simulink model "Tricopter_Controlled_development"  (R2015a)
settings: Solver=ode2  SolverMode=SingleTasking  StartTime=0.0  StopTime=inf  FixedStep=T_sim  RelTol=1e-3
values from neighbouring files (symbols this model uses):
  A_l_max_x = sqrt( (A_z_max)^2  -  g^2  )    [Run3Copter.m]
  A_l_max_y = g*tand(15)    [Run3Copter.m]
  A_x = 0.015    [SetupComplete.m]
  A_y = A_x    (= 0.015)    [SetupComplete.m]
  A_z = 0.16    [SetupComplete.m]
  A_z_max = Max_Thrust*3/m    [Run3Copter.m]
  Alt_0 = input(' Give the initial altitude (m): ')    [Run3Copter.m]
  C_x = 1.2    [SetupComplete.m]
  C_y = C_x    (= 1.2)    [SetupComplete.m]
  C_z = 2.2    [SetupComplete.m]
  CG_0 = [0,0,0.02]'    [SetupComplete.m]
  epsilon = 0.01    [Run3Copter.m]
  eta_23 = deg2rad(-1.3)    [Run3Copter.m]
  g = 9.81    [SetupComplete.m]
  h = 0.08    [SetupComplete.m]
  h_M = 0.064    [SetupComplete.m]
  I_BAC_0 = [ Ix,0,Ixz;0,Iy,0;Ixz,0,Iz]    [SetupComplete.m]
  Initial_Omegas = Omega_hover    [Run3Copter.m]
  Initial_Torques = Torque_hover    [Run3Copter.m]
  Ix = 0.103    [SetupComplete.m]
  Iy = 0.147    [SetupComplete.m]
  Iz = 0.237    [SetupComplete.m]
  l = 0.345    [SetupComplete.m]
  l_arm = 0.264    [SetupComplete.m]
  latitude = 52.071118    [Run3Copter.m]
  longitude = -0.627404    [Run3Copter.m]
  m = 3.51    [SetupComplete.m]
  m_0 = 2.61    [SetupComplete.m]
  m_M = 0.300    (= 0.3)    [SetupComplete.m]
  rho = 1.15    [SetupComplete.m]
  Rotation_sign = [ 1,-1,-1]    [SetupComplete.m]
  T_ctrl = 0.02    [Run3Copter.m]
  T_sim = 0.01    [Run3Copter.m]
  throtle_1 = 0*0.745    (= 0)    [Run3Copter.m]
  throtle_23 = throtle_1/cos(eta_23)    [Run3Copter.m]
  v_i0 = sqrt( 1/3*m*g/(2*rho*pi*R^2)  )    [SetupComplete.m]
undefined symbols (not defined in the file or in its folder): DOWN_0, EAST_0, Newton, NORTH_0, P_0, Q_0, R_0, Raphson, U_0, V_0, W_0
libraries: Adaptive_FaultTolerantControl x30, XXCopter_Control x23, simulink_extras x17, XXCopter x5, simulink x2, qcatlib x1, XXCopter_C x1
(part 3 of 4)

== system Tricopter_Controlled_development/TriCopter FCS development/Inner Controller/PI Controller/keep -pi//pi2 ==
  in (rad) : Inport
  Constant : Constant  Value=180
  Constant2 : Constant  Value=360
  Gain : Gain  Gain=360
  Math Function2 : Math  Operator=rem  SaturateOnIntegerOverflow=on
  Product : Product  Inputs=*/  RndMeth=Zero
  Rounding Function : Rounding  Operator=fix
  Sum2 : Sum  Inputs=|-+
  deg2rad1 : Gain  Gain=pi/180  SaturateOnIntegerOverflow=on  OutDataTypeStr=Inherit: Same as input  ParamDataTypeStr=Inherit: Same as input
  rad2deg : Gain  Gain=180/pi  SaturateOnIntegerOverflow=on  OutDataTypeStr=Inherit: Same as input  ParamDataTypeStr=Inherit: Same as input
  out (rad) : Outport
  wires:
  deg2rad1/1 -> out (rad)/1
  Sum2/1 -> deg2rad1/1
  Math Function2/1 -> Sum2/2, Product/1
  Constant2/1 -> Math Function2/2
  rad2deg/1 -> Math Function2/1
  Gain/1 -> Sum2/1
  Rounding Function/1 -> Gain/1
  Product/1 -> Rounding Function/1
  Constant/1 -> Product/2
  in (rad)/1 -> rad2deg/1

== system Tricopter_Controlled_development/TriCopter FCS development/Inner Controller/PI Controller/keep -pi//pi3 ==
  in (rad) : Inport
  Constant : Constant  Value=180
  Constant2 : Constant  Value=360
  Gain : Gain  Gain=360
  Math Function2 : Math  Operator=rem  SaturateOnIntegerOverflow=on
  Product : Product  Inputs=*/  RndMeth=Zero
  Rounding Function : Rounding  Operator=fix
  Sum2 : Sum  Inputs=|-+
  deg2rad1 : Gain  Gain=pi/180  SaturateOnIntegerOverflow=on  OutDataTypeStr=Inherit: Same as input  ParamDataTypeStr=Inherit: Same as input
  rad2deg : Gain  Gain=180/pi  SaturateOnIntegerOverflow=on  OutDataTypeStr=Inherit: Same as input  ParamDataTypeStr=Inherit: Same as input
  out (rad) : Outport
  wires:
  in (rad)/1 -> rad2deg/1
  Constant/1 -> Product/2
  Product/1 -> Rounding Function/1
  Rounding Function/1 -> Gain/1
  Gain/1 -> Sum2/1
  rad2deg/1 -> Math Function2/1
  Constant2/1 -> Math Function2/2
  Math Function2/1 -> Product/1, Sum2/2
  Sum2/1 -> deg2rad1/1
  deg2rad1/1 -> out (rad)/1

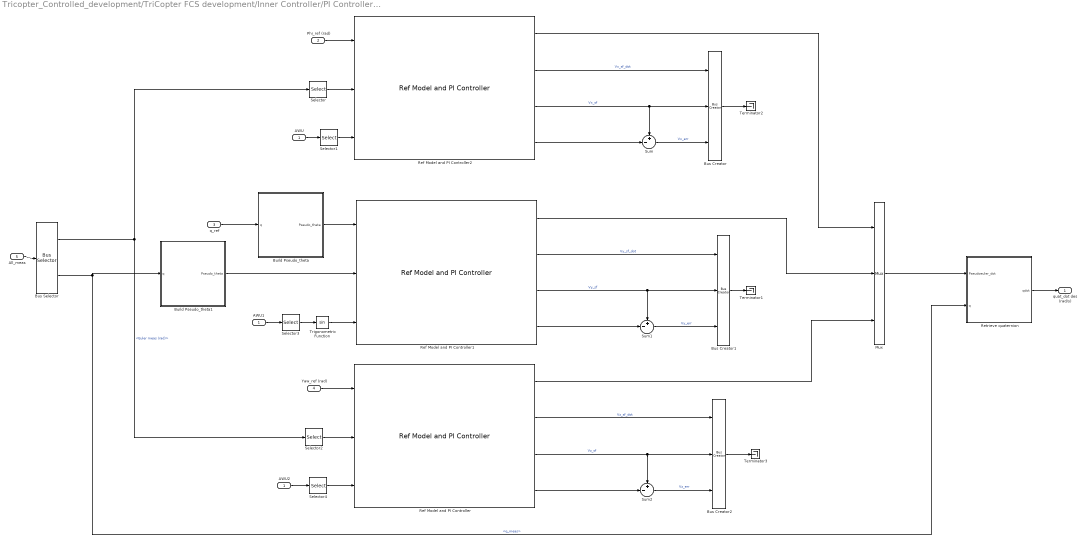
== system Tricopter_Controlled_development/TriCopter FCS development/Inner Controller/PI Controller Quaternions/Attitude Controller ==
  AWU : Inport
  Phi_ref (rad) : Inport  Port=2
  q_ref : Inport  Port=3
  Yaw_ref (rad) : Inport  Port=4
  All_meas : Inport  Port=5
  AWU1 : InportShadow
  AWU2 : InportShadow
  Build Pseudo_theta : MATLAB Function  TreatAsAtomicUnit=on
  Build Pseudo_theta1 : MATLAB Function  TreatAsAtomicUnit=on
  Bus Creator : BusCreator  Inputs=3
  Bus Creator1 : BusCreator  Inputs=3
  Bus Creator2 : BusCreator  Inputs=3
  Bus Selector : BusSelector  OutputSignals=Meas.Euler meas (rad),Meas.q_meas
  Mux : Mux  Inputs=3
  Ref Model and PI Controller : Adaptive_FaultTolerantControl/Ref Model and PI Controller  delta=0  tau=2  y_i=0  K_f=0  K_a=1  Con_way=pro  omega_n=4  xi=0.5  Z1=-30  K_b=2  f_i=0.15  f_c=1
  Ref Model and PI Controller1 : Adaptive_FaultTolerantControl/Ref Model and PI Controller  delta=0  tau=1.5  y_i=0  K_f=0  K_a=1  Con_way=pro  omega_n=4  xi=0.5  Z1=-30  K_b=1.2  f_i=0.1  f_c=1
  Ref Model and PI Controller2 : Adaptive_FaultTolerantControl/Ref Model and PI Controller  delta=0  tau=1.5  y_i=0  K_f=0  K_a=1  Con_way=pro  omega_n=4  xi=0.5  Z1=-30  K_b=1.5  f_i=0.1  f_c=1
  Retrieve quaternion : MATLAB Function  TreatAsAtomicUnit=on
  Selector : Selector  InputPortWidth=3
  Selector1 : Selector  InputPortWidth=3
  Selector2 : Selector  InputPortWidth=3  Indices=3
  Selector3 : Selector  InputPortWidth=3  Indices=2
  Selector4 : Selector  InputPortWidth=3  Indices=3
  Sum : Sum  Inputs=+-|
  Sum1 : Sum  Inputs=+-|
  Sum2 : Sum  Inputs=+-|
  Terminator1 : Terminator
  Terminator2 : Terminator
  Terminator3 : Terminator
  Trigonometric Function : Trigonometry
  quat_dot des (rad/s) : Outport
  wires:
  Ref Model and PI Controller/4 -> Sum2/2
  Sum2/1 -> Bus Creator2/3  "Vz_err"
  Ref Model and PI Controller/3 -> Bus Creator2/2, Sum2/1  "Vz_sf"
  Ref Model and PI Controller/2 -> Bus Creator2/1  "Vz_sf_dot"
  Ref Model and PI Controller1/4 -> Sum1/2
  Sum1/1 -> Bus Creator1/3  "Vy_err"
  Ref Model and PI Controller1/3 -> Bus Creator1/2, Sum1/1  "Vy_sf"
  Ref Model and PI Controller1/2 -> Bus Creator1/1  "Vy_sf_dot"
  Ref Model and PI Controller2/4 -> Sum/2
  Bus Creator2/1 -> Terminator3/1
  Bus Creator1/1 -> Terminator1/1
  Bus Creator/1 -> Terminator2/1
  Sum/1 -> Bus Creator/3  "Vx_err"
  Ref Model and PI Controller2/3 -> Bus Creator/2, Sum/1  "Vx_sf"
  Ref Model and PI Controller2/2 -> Bus Creator/1  "Vx_sf_dot"
  Yaw_ref (rad)/1 -> Ref Model and PI Controller/1
  Selector/1 -> Ref Model and PI Controller2/2
  Bus Selector/2 -> Retrieve quaternion/2(q), Build Pseudo_theta1/1(q)  "<q_meas>"
  All_meas/1 -> Bus Selector/1
  q_ref/1 -> Build Pseudo_theta/1(q)
  Phi_ref (rad)/1 -> Ref Model and PI Controller2/1
  Retrieve quaternion/1(qdot) -> quat_dot des (rad/s)/1
  Ref Model and PI Controller2/1 -> Mux/1
  Ref Model and PI Controller/1 -> Mux/3
  Ref Model and PI Controller1/1 -> Mux/2
  Mux/1 -> Retrieve quaternion/1(Pseudoeuler_dot)
  Selector2/1 -> Ref Model and PI Controller/2
  Bus Selector/1 -> Selector2/1, Selector/1  "<Euler meas (rad)>"
  Build Pseudo_theta1/1(Pseudo_theta) -> Ref Model and PI Controller1/2
  Build Pseudo_theta/1(Pseudo_theta) -> Ref Model and PI Controller1/1
  Selector1/1 -> Ref Model and PI Controller2/3
  AWU/1 -> Selector1/1
  AWU1/1 -> Selector3/1
  AWU2/1 -> Selector4/1
  Selector4/1 -> Ref Model and PI Controller/3
  Selector3/1 -> Trigonometric Function/1
  Trigonometric Function/1 -> Ref Model and PI Controller1/3

== system Tricopter_Controlled_development/TriCopter FCS development/Inner Controller/PI Controller Quaternions/Body Rates Controller ==
  p_ref : Inport
  q_ref : Inport  Port=2
  r_ref : Inport  Port=3
  All_meas : Inport  Port=4
  Bus Creator : BusCreator
  Bus Creator1 : BusCreator
  Bus Creator2 : BusCreator
  Bus Selector : BusSelector  OutputSignals=Meas.omega_b meas (rad/s)
  Mux : Mux  Inputs=3
  Ref Model and P Controller p : Adaptive_FaultTolerantControl/Ref Model and P Controller  tau=0.7  y_i=0  K_f=0.7  K_b=6
  Ref Model and P Controller q : Adaptive_FaultTolerantControl/Ref Model and P Controller  tau=0.7  y_i=0  K_f=0.7  K_b=6
  Ref Model and P Controller r : Adaptive_FaultTolerantControl/Ref Model and P Controller  tau=1.5  y_i=0  K_f=0.7  K_b=1.5
  Selector : Selector  InputPortWidth=3
  Selector1 : Selector  InputPortWidth=3  Indices=2
  Selector2 : Selector  InputPortWidth=3  Indices=3
  Sum : Sum  Inputs=+-|
  Sum1 : Sum  Inputs=+-|
  Sum2 : Sum  Inputs=+-|
  Terminator1 : Terminator
  Terminator2 : Terminator
  Terminator3 : Terminator
  Angular acc des (rad/s^2) : Outport
  wires:
  Ref Model and P Controller r/5 -> Bus Creator2/4  "K_b_r"
  Ref Model and P Controller r/4 -> Sum2/2
  Sum2/1 -> Bus Creator2/3  "r_err"
  Ref Model and P Controller r/3 -> Bus Creator2/2, Sum2/1  "r_sf"
  Ref Model and P Controller r/2 -> Bus Creator2/1  "r_sf_dot"
  Ref Model and P Controller q/5 -> Bus Creator1/4  "K_b_q"
  Ref Model and P Controller q/4 -> Sum1/2
  Sum1/1 -> Bus Creator1/3  "q_err"
  Ref Model and P Controller q/3 -> Bus Creator1/2, Sum1/1  "q_sf"
  Ref Model and P Controller q/2 -> Bus Creator1/1  "q_sf_dot"
  Ref Model and P Controller p/5 -> Bus Creator/4  "K_b_p"
  Ref Model and P Controller p/4 -> Sum/2
  Selector2/1 -> Ref Model and P Controller r/2
  Bus Creator2/1 -> Terminator3/1
  Bus Creator1/1 -> Terminator1/1
  Bus Creator/1 -> Terminator2/1
  Sum/1 -> Bus Creator/3  "p_err"
  Ref Model and P Controller p/3 -> Bus Creator/2, Sum/1  "p_sf"
  Ref Model and P Controller p/2 -> Bus Creator/1  "p_sf_dot"
  r_ref/1 -> Ref Model and P Controller r/1
  Selector1/1 -> Ref Model and P Controller q/2
  q_ref/1 -> Ref Model and P Controller q/1
  Mux/1 -> Angular acc des (rad/s^2)/1
  Selector/1 -> Ref Model and P Controller p/2
  p_ref/1 -> Ref Model and P Controller p/1
  Bus Selector/1 -> Selector2/1, Selector1/1, Selector/1  "<omega_b meas (rad/s)>"
  All_meas/1 -> Bus Selector/1
  Ref Model and P Controller r/1 -> Mux/3
  Ref Model and P Controller q/1 -> Mux/2
  Ref Model and P Controller p/1 -> Mux/1

== system Tricopter_Controlled_development/TriCopter FCS development/Inner Controller/PI Controller Quaternions/Limits in Ang accel ==
  note: Here it is assumed that at all time every prop is generating m*g/3 newtons of force . It is conservative?
  Ang Ace des : Inport
  Euler meas : Inport  Port=2
  Limis eval : MATLAB Function  TreatAsAtomicUnit=on
  Saturation Dynamic : simulink/Discontinuities/Saturation Dynamic  OutMin=[]  OutMax=[]  OutDataTypeStr=Inherit: Same as second input  OutDataType=fixdt(1, 16)  OutScaling=2^-10  DoSatur=off
  ang Ace des : Outport
  wires:
  Limis eval/1(Limit_up) -> Saturation Dynamic/1
  Limis eval/2(Limit_down) -> Saturation Dynamic/3
  Euler meas/1 -> Limis eval/2(euler_ang)
  Ang Ace des/1 -> Saturation Dynamic/2, Limis eval/1(Ang_Accel)
  Saturation Dynamic/1 -> ang Ace des/1

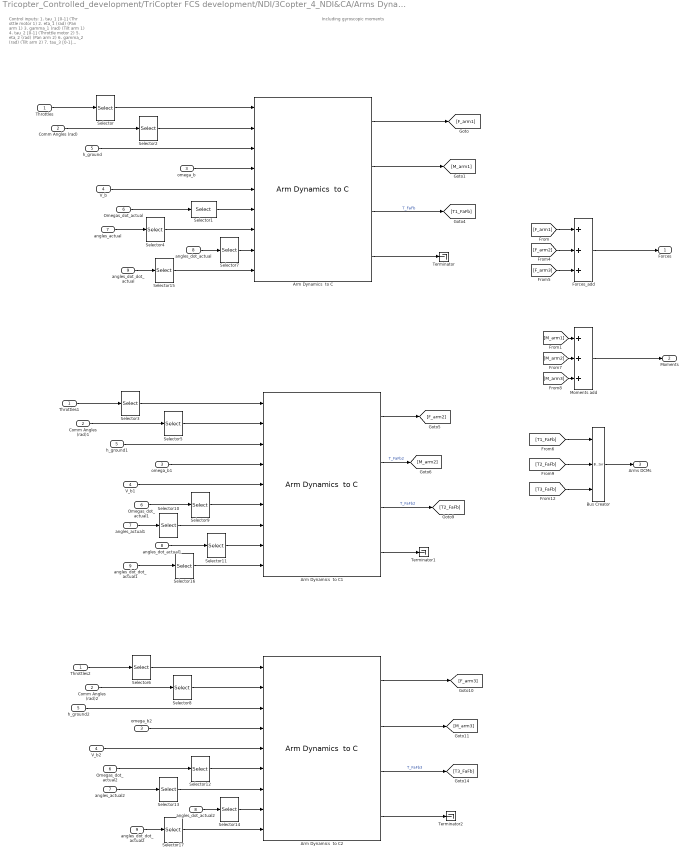
== system Tricopter_Controlled_development/TriCopter FCS development/NDI/3Copter_4_NDI&CA/Arms Dynamics: Forces and Moments ==
  note: Including gyroscopic moments
  note: Control inputs:
      | 1. tau_1 [0-1] (Thr ottle motor 1)
      | 2. eta_1 (rad)  (Pan arm 1)
      | 3. gamma_1 (rad)  (Tilt arm 1)
      |
      | 4. tau_2 [0-1] (Throttle motor 2)
      | 5. eta_2 (rad)  (Pan arm 2)
      | 6. gamma_2 (rad)  (Tilt arm 2)
      |
      | 7. tau_3 [0-1] (Throttle motor 3)
      | 8. eta_3 (rad)  (Pan arm  3)
      | 9. gamma_3 (rad)  (Tilt arm 3)
  Throttles : Inport
  Comm Angles (rad) : Inport  Port=2
  omega_b : Inport  Port=3
  V_b : Inport  Port=4
  h_ground : Inport  Port=5
  Omegas_dot_actual : Inport  Port=6
  angles_actual : Inport  Port=7
  angles_dot_actual : Inport  Port=8
  angles_dot_dot_actual : Inport  Port=9
  Arm Dynamics  to C : XXCopter_Control/Arm Dynamics  to C  Rot_sign=Rotation_sign(1)  arm_hub_pos=l*[1;0;0]  Arm_axis=[l_arm;0;0]  arm_num=1  eta_dir=[1;0;0]  gamma_dir=[0;1;0]  J_T=J_T  J_FA=J_FA  h=h  switch_val=direct_feedforward  omega_n=30  xi=1.4  eta_inf_lim=deg2rad(-180)  eta_sup_lim=deg2rad(180)  gamma_inf_lim=deg2rad(-90)  gamma_sup_lim=deg2rad(15)
      link override Aerodynamics Propeller/2D vec norm: SourceBlock=XXCopter_Control/2D vec norm
      link override Aerodynamics Propeller/2D vec norm1: SourceBlock=XXCopter_Control/2D vec norm
      link override "Aerodynamics Propeller/Aero Forces and Moments ": SourceBlock=XXCopter_Control/Aero Forces and Moments
      link override Aerodynamics Propeller/Aero Forces and Moments /Normalize 2D vector: SourceBlock=XXCopter_Control/Normalize 2D vector
      link override Aerodynamics Propeller/Aero Forces and Moments /Normalize 2D vector/2D vec norm: SourceBlock=XXCopter_Control/2D vec norm
      link override Arms Kinematics  to C: SourceBlock="XXCopter_Control/Arms Kinematics  to C"
      link override ESC+Motor Dynamcis  to C: SourceBlock="XXCopter_Control/ESC+Motor Dynamcis  to C"
      link override Gyroscopic Moments  to C: SourceBlock="XXCopter_Control/Gyroscopic Moments  to C"
      link override Servos Dynamics  to C: SourceBlock="XXCopter_Control/Servos Dynamics  to C"
  Arm Dynamics  to C1 : XXCopter_Control/Arm Dynamics  to C  Rot_sign=Rotation_sign(2)  arm_hub_pos=l*[-1/2;sqrt(3)/2;0]  Arm_axis=[0;l_arm;0]  arm_num=2  eta_dir=[0;1;0]  gamma_dir=[1;0;0]  J_T=J_T  J_FA=J_FA  h=h  switch_val=direct_feedforward  omega_n=30  xi=1.4  eta_inf_lim=deg2rad(-180)  eta_sup_lim=deg2rad(180)  gamma_inf_lim=deg2rad(-15)  gamma_sup_lim=deg2rad(90)
      link override Aerodynamics Propeller/Aero Forces and Moments /Normalize 2D vector/2D vec norm: SourceBlock=XXCopter_Control/2D vec norm
  Arm Dynamics  to C2 : XXCopter_Control/Arm Dynamics  to C  Rot_sign=Rotation_sign(3)  arm_hub_pos=l*[-1/2;-sqrt(3)/2;0]  Arm_axis=[0;-l_arm;0]  arm_num=3  eta_dir=[0;1;0]  gamma_dir=[1;0;0]  J_T=J_T  J_FA=J_FA  h=h  switch_val=direct_feedforward  omega_n=30  xi=1.4  eta_inf_lim=deg2rad(-180)  eta_sup_lim=deg2rad(180)  gamma_inf_lim=deg2rad(-90)  gamma_sup_lim=deg2rad(15)
  Bus Creator : BusCreator  Inputs=3
  Comm Angles (rad)1 : InportShadow  Port=2
  Comm Angles (rad)2 : InportShadow  Port=2
  Forces_add : Sum  Inputs=+++
  Moments add : Sum  Inputs=+++
  Omegas_dot_actual1 : InportShadow  Port=6
  Omegas_dot_actual2 : InportShadow  Port=6
  Selector : Selector  IndexMode=Zero-based  InputPortWidth=3  Indices=0
  Selector1 : Selector  IndexMode=Zero-based  InputPortWidth=3  Indices=0
  Selector{5,10..11,16} (4 alike) : Selector  IndexMode=Zero-based  InputPortWidth=6  Indices=[2,3]
  Selector12 : Selector  IndexMode=Zero-based  InputPortWidth=3  Indices=2
  Selector{8,13..14,17} (4 alike) : Selector  IndexMode=Zero-based  InputPortWidth=6  Indices=[4,5]
  Selector{2,4,7,15} (4 alike) : Selector  IndexMode=Zero-based  InputPortWidth=6  Indices=[0,1]
  Selector3 : Selector  IndexMode=Zero-based  InputPortWidth=3
  Selector6 : Selector  IndexMode=Zero-based  InputPortWidth=3  Indices=2
  Selector9 : Selector  IndexMode=Zero-based  InputPortWidth=3
  Terminator : Terminator
  Terminator1 : Terminator
  Terminator2 : Terminator
  Throttles1 : InportShadow
  Throttles2 : InportShadow
  V_b1 : InportShadow  Port=4
  V_b2 : InportShadow  Port=4
  angles_actual1 : InportShadow  Port=7
  angles_actual2 : InportShadow  Port=7
  angles_dot_actual1 : InportShadow  Port=8
  angles_dot_actual2 : InportShadow  Port=8
  angles_dot_dot_actual1 : InportShadow  Port=9
  angles_dot_dot_actual2 : InportShadow  Port=9
  h_ground1 : InportShadow  Port=5
  h_ground2 : InportShadow  Port=5
  omega_b1 : InportShadow  Port=3
  omega_b2 : InportShadow  Port=3
  Forces : Outport
  Moments : Outport  Port=2
  Arms DCMs : Outport  Port=3
  wires:
  Selector14/1 -> Arm Dynamics  to C2/8
  angles_actual2/1 -> Selector13/1
  angles_dot_actual2/1 -> Selector14/1
  Selector13/1 -> Arm Dynamics  to C2/7
  Selector12/1 -> Arm Dynamics  to C2/6
  Omegas_dot_actual2/1 -> Selector12/1
  Selector11/1 -> Arm Dynamics  to C1/8
  angles_actual1/1 -> Selector10/1
  angles_dot_actual1/1 -> Selector11/1
  Selector10/1 -> Arm Dynamics  to C1/7
  Selector9/1 -> Arm Dynamics  to C1/6
  Omegas_dot_actual1/1 -> Selector9/1
  Selector7/1 -> Arm Dynamics  to C/8
  angles_dot_actual/1 -> Selector7/1
  Selector4/1 -> Arm Dynamics  to C/7
  angles_actual/1 -> Selector4/1
  Selector1/1 -> Arm Dynamics  to C/6
  Omegas_dot_actual/1 -> Selector1/1
  [T3_FaFb] -> Bus Creator/3
  [T2_FaFb] -> Bus Creator/2
  [T1_FaFb] -> Bus Creator/1
  Bus Creator/1 -> Arms DCMs/1
  Arm Dynamics  to C1/2 -> [M_arm2]  "T_FaFb2"
  Arm Dynamics  to C1/1 -> [F_arm2]
  Arm Dynamics  to C2/4 -> Terminator2/1
  Arm Dynamics  to C1/4 -> Terminator1/1
  Arm Dynamics  to C/4 -> Terminator/1
  Arm Dynamics  to C2/3 -> [T3_FaFb]  "T_FaFb3"
  Comm Angles (rad)2/1 -> Selector8/1
  Selector8/1 -> Arm Dynamics  to C2/2
  omega_b2/1 -> Arm Dynamics  to C2/4
  Arm Dynamics  to C2/2 -> [M_arm3]
  Arm Dynamics  to C2/1 -> [F_arm3]
  h_ground2/1 -> Arm Dynamics  to C2/3
  V_b2/1 -> Arm Dynamics  to C2/5
  Selector6/1 -> Arm Dynamics  to C2/1
  Throttles2/1 -> Selector6/1
  Arm Dynamics  to C1/3 -> [T2_FaFb]  "T_FaFb2"
  Comm Angles (rad)1/1 -> Selector5/1
  Selector5/1 -> Arm Dynamics  to C1/2
  omega_b1/1 -> Arm Dynamics  to C1/4
  h_ground1/1 -> Arm Dynamics  to C1/3
  V_b1/1 -> Arm Dynamics  to C1/5
  Selector3/1 -> Arm Dynamics  to C1/1
  Throttles1/1 -> Selector3/1
  Arm Dynamics  to C/3 -> [T1_FaFb]  "T_FaFb"
  Comm Angles (rad)/1 -> Selector2/1
  Selector2/1 -> Arm Dynamics  to C/2
  [M_arm2] -> Moments add/2
  [M_arm3] -> Moments add/3
  [F_arm3] -> Forces_add/3
  [F_arm2] -> Forces_add/2
  omega_b/1 -> Arm Dynamics  to C/4
  [M_arm1] -> Moments add/1
  [F_arm1] -> Forces_add/1
  Arm Dynamics  to C/2 -> [M_arm1]
  Arm Dynamics  to C/1 -> [F_arm1]
  h_ground/1 -> Arm Dynamics  to C/3
  Moments add/1 -> Moments/1
  Forces_add/1 -> Forces/1
  V_b/1 -> Arm Dynamics  to C/5
  Selector/1 -> Arm Dynamics  to C/1
  Throttles/1 -> Selector/1
  angles_dot_dot_actual/1 -> Selector15/1
  Selector15/1 -> Arm Dynamics  to C/9
  angles_dot_dot_actual1/1 -> Selector16/1
  Selector16/1 -> Arm Dynamics  to C1/9
  angles_dot_dot_actual2/1 -> Selector17/1
  Selector17/1 -> Arm Dynamics  to C2/9

== system Tricopter_Controlled_development/TriCopter FCS development/NDI/3Copter_4_NDI&CA/Gradient ==
  note: Control inputs:
      | 1. tau_1 [0-1] (Thr ottle motor 1)
      | 2. eta_1 (rad)  (Pan arm 1)
      | 3. gamma_1 (rad)  (Tilt arm 1)
      |
      | 4. tau_2 [0-1] (Throttle motor 2)
      | 5. eta_2 (rad)  (Pan arm 2)
      | 6. gamma_2 (rad)  (Tilt arm 2)
      |
      | 7. tau_3 [0-1] (Throttle motor 3)
      | 8. eta_3 (rad)  (Pan arm  3)
      | 9. gamma_3 (rad)  (Tilt arm 3)
  "Control Inputs(rad) " : Inport  Partition=on  PartitionDimension=1  PartitionWidth=9
  h : Inport  Port=2  Partition=off
  Vb : Inport  Port=3  Partition=off
  omega_b : Inport  Port=4  Partition=off
  Omegas_dot_actual : Inport  Port=5  Partition=off
  angles_actual : Inport  Port=6  Partition=off
  angles_dot_actual : Inport  Port=7  Partition=off
  angles_dot_dot_actual : Inport  Port=8  Partition=off
  F_g : Inport  Port=9  Partition=off
  M_g : Inport  Port=10  Partition=off
  Add : Sum
  Add1 : Sum
  Arms Dynamics: Forces and Moments : Subsystem  TreatAsAtomicUnit=on
  Equivalent Throttle : Product  Inputs=**
  For Each : ForEach  DisableCoverage=on  IndexMode=One-based
  Mux : Mux  Inputs=[3,3]
  Reference batrery level (V) : Constant  Value=16
  Signal Specification : SignalSpecification  Dimensions=[6,1]
  Terminator : Terminator
  Throttles : Selector  IndexMode=Zero-based  InputPortWidth=9  Indices=[0,3,6]
  "angles " : Selector  IndexMode=Zero-based  InputPortWidth=9  Indices=[1,2,4,5,7,8]
  Forces_Moments : Outport  ConcatenationDimension=2
  wires:
  Signal Specification/1 -> Forces_Moments/1
  Mux/1 -> Signal Specification/1
  Add1/1 -> Mux/2
  Add/1 -> Mux/1
  M_g/1 -> Add1/2
  F_g/1 -> Add/2
  angles_dot_actual/1 -> Arms Dynamics: Forces and Moments/8(angles_dot_actual)
  Omegas_dot_actual/1 -> Arms Dynamics: Forces and Moments/6(Omegas_dot_actual)
  Reference batrery level (V)/1 -> Equivalent Throttle/1
  Equivalent Throttle/1 -> Arms Dynamics: Forces and Moments/1(Throttles)
  "Control Inputs(rad) "/1 -> "angles "/1, Throttles/1
  Throttles/1 -> Equivalent Throttle/2
  Arms Dynamics: Forces and Moments/1(Forces) -> Add/1
  h/1 -> Arms Dynamics: Forces and Moments/5(h_ground)
  omega_b/1 -> Arms Dynamics: Forces and Moments/3(omega_b)
  angles_actual/1 -> Arms Dynamics: Forces and Moments/7(angles_actual)
  "angles "/1 -> Arms Dynamics: Forces and Moments/2(Comm Angles (rad))
  angles_dot_dot_actual/1 -> Arms Dynamics: Forces and Moments/9(angles_dot_dot_actual)
  Arms Dynamics: Forces and Moments/2(Moments) -> Add1/1
  Arms Dynamics: Forces and Moments/3(Arms DCMs) -> Terminator/1
  Vb/1 -> Arms Dynamics: Forces and Moments/4(V_b)

== system Tricopter_Controlled_development/TriCopter FCS development/NDI/3Copter_4_NDI&CA/Mass Properties ==
  Arms DCMs : Inport
  CG_0 : Inport  Port=2
  m_0 : Inport  Port=3
  m : Inport  Port=4
  m_M : Inport  Port=5
  I_BAC_0 : Inport  Port=6
  Arm Inertia : MATLAB Function  TreatAsAtomicUnit=on
  Bus Selector : BusSelector  OutputSignals=T_FaFb,T_FaFb2,T_FaFb3
  CG position : Sum
  Divide : Product  Inputs=*/
  Divide1 : Product  Inputs=**
  Divide2 : Product  Inputs=/*
  Divide3 : Product  Inputs=**
  Motors Pos sum : Sum  Inputs=+++
  Total I_BAC : Sum
  I_BAC : Outport
  CG : Outport  Port=2
  wires:
  Arm Inertia/2(r1_M) -> Motors Pos sum/3
  I_BAC_0/1 -> Total I_BAC/1
  Arm Inertia/1(I_M) -> Total I_BAC/2
  Arm Inertia/4(r3_M) -> Motors Pos sum/1
  Arm Inertia/3(r2_M) -> Motors Pos sum/2
  Divide3/1 -> CG position/2
  Divide2/1 -> Divide3/2
  Motors Pos sum/1 -> Divide3/1
  Divide1/1 -> CG position/1
  CG position/1 -> CG/1
  m_M/1 -> Divide2/2
  Divide/1 -> Divide1/2
  CG_0/1 -> Divide1/1
  m/1 -> Divide2/1, Divide/2
  m_0/1 -> Divide/1
  Total I_BAC/1 -> I_BAC/1
  Bus Selector/1 -> Arm Inertia/1(T1_FAFb)  "<T_FaFb>"
  Bus Selector/2 -> Arm Inertia/2(T2_FAFb)  "<T_FaFb2>"
  Bus Selector/3 -> Arm Inertia/3(T3_FAFb)  "<T_FaFb3>"
  Arms DCMs/1 -> Bus Selector/1

== system Tricopter_Controlled_development/TriCopter FCS development/Outer Controller/Overactuated P Controller/Position Controller ==
  AWU : Inport
  X_e_x_ref : Inport  Port=2
  X_e_y_ref : Inport  Port=3
  X_e_z_ref : Inport  Port=4
  All_meas : Inport  Port=5
  AWU1 : InportShadow
  AWU2 : InportShadow
  Bus Creator : BusCreator  Inputs=3
  Bus Creator1 : BusCreator  Inputs=3
  Bus Creator2 : BusCreator  Inputs=3
  Bus Selector : BusSelector  OutputSignals=Meas.Pos meas (m)
  Mux : Mux  Inputs=3
  Ref Model and PI Controller : Adaptive_FaultTolerantControl/Ref Model and PI Controller  delta=0  tau=3  y_i=-Alt_0  K_f=0  K_a=1  Con_way=pro  omega_n=4  xi=0.5  Z1=-30  K_b=1.2  f_i=0.07  f_c=1
  Ref Model and PI Controller1 : Adaptive_FaultTolerantControl/Ref Model and PI Controller  delta=0  tau=5  y_i=0  K_f=0  K_a=1  Con_way=pro  omega_n=4  xi=0.5  Z1=-30  K_b=1.1  f_i=0.07  f_c=1
  Ref Model and PI Controller2 : Adaptive_FaultTolerantControl/Ref Model and PI Controller  delta=0  tau=5  y_i=0  K_f=0  K_a=1  Con_way=pro  omega_n=4  xi=0.5  Z1=-30  K_b=1.1  f_i=0.07  f_c=1
  Selector : Selector  InputPortWidth=3
  Selector1 : Selector  InputPortWidth=3  Indices=2
  Selector2 : Selector  InputPortWidth=3  Indices=3
  Selector3 : Selector  InputPortWidth=3
  Selector4 : Selector  InputPortWidth=3  Indices=2
  Selector5 : Selector  InputPortWidth=3  Indices=3
  Sum : Sum  Inputs=+-|
  Sum1 : Sum  Inputs=+-|
  Sum2 : Sum  Inputs=+-|
  Terminator1 : Terminator
  Terminator2 : Terminator
  Terminator3 : Terminator
  Ve des (m/s) : Outport
  wires:
  All_meas/1 -> Bus Selector/1
  Bus Selector/1 -> Selector1/1, Selector/1, Selector2/1  "<Pos meas (m)>"
  X_e_x_ref/1 -> Ref Model and PI Controller2/1
  Selector/1 -> Ref Model and PI Controller2/2
  Ref Model and PI Controller2/1 -> Mux/1
  Mux/1 -> Ve des (m/s)/1
  X_e_y_ref/1 -> Ref Model and PI Controller1/1
  Selector1/1 -> Ref Model and PI Controller1/2
  X_e_z_ref/1 -> Ref Model and PI Controller/1
  Ref Model and PI Controller1/1 -> Mux/2
  Ref Model and PI Controller/1 -> Mux/3
  Ref Model and PI Controller2/2 -> Bus Creator/1  "X_ex_sf_dot"
  Ref Model and PI Controller2/3 -> Bus Creator/2, Sum/1  "X_ex_sf"
  Sum/1 -> Bus Creator/3  "X_ex_err"
  Bus Creator/1 -> Terminator2/1
  Bus Creator1/1 -> Terminator1/1
  Bus Creator2/1 -> Terminator3/1
  Selector2/1 -> Ref Model and PI Controller/2
  Ref Model and PI Controller2/4 -> Sum/2
  Ref Model and PI Controller1/2 -> Bus Creator1/1  "X_ey_sf_dot"
  Ref Model and PI Controller1/3 -> Sum1/1, Bus Creator1/2  "X_e_y_sf"
  Sum1/1 -> Bus Creator1/3  "X_ey_err"
  Ref Model and PI Controller1/4 -> Sum1/2
  Ref Model and PI Controller/2 -> Bus Creator2/1  "X_ez_sf_dot"
  Ref Model and PI Controller/3 -> Sum2/1, Bus Creator2/2  "X_ez_sf"
  Sum2/1 -> Bus Creator2/3  "X_ez_err"
  Ref Model and PI Controller/4 -> Sum2/2
  Selector3/1 -> Ref Model and PI Controller2/3
  AWU/1 -> Selector3/1
  Selector4/1 -> Ref Model and PI Controller1/3
  AWU1/1 -> Selector4/1
  AWU2/1 -> Selector5/1
  Selector5/1 -> Ref Model and PI Controller/3

== system Tricopter_Controlled_development/TriCopter FCS development/Outer Controller/Overactuated P Controller/Velocity Controller ==
  Vyaw_x_ref : Inport
  Vyaw_y_ref : Inport  Port=2
  Vyaw_z_ref : Inport  Port=3
  V_yaw_meas : Inport  Port=4
  Bus Creator : BusCreator
  Bus Creator1 : BusCreator
  Bus Creator2 : BusCreator
  Mux : Mux  Inputs=3
  Ref Model and P Controller p : Adaptive_FaultTolerantControl/Ref Model and P Controller  tau=1.7  y_i=0  K_f=0.5  K_b=6
  Ref Model and P Controller q : Adaptive_FaultTolerantControl/Ref Model and P Controller  tau=1.7  y_i=0  K_f=0.5  K_b=6
  Ref Model and P Controller r : Adaptive_FaultTolerantControl/Ref Model and P Controller  tau=1  y_i=0  K_f=0.4  K_b=8
  Selector : Selector  InputPortWidth=3
  Selector1 : Selector  InputPortWidth=3  Indices=2
  Selector2 : Selector  InputPortWidth=3  Indices=3
  Sum : Sum  Inputs=+-|
  Sum1 : Sum  Inputs=+-|
  Sum2 : Sum  Inputs=+-|
  Terminator1 : Terminator
  Terminator2 : Terminator
  Terminator3 : Terminator
  Acc_yaw des (m/s) : Outport
  wires:
  Ref Model and P Controller r/5 -> Bus Creator2/4  "K_b_Ve_z"
  Ref Model and P Controller r/4 -> Sum2/2
  Sum2/1 -> Bus Creator2/3  "Vez_err"
  Ref Model and P Controller r/3 -> Bus Creator2/2, Sum2/1  "Vez_sf"
  Ref Model and P Controller r/2 -> Bus Creator2/1  "Vez_sf_dot"
  Ref Model and P Controller q/5 -> Bus Creator1/4  "K_b_Vey"
  Ref Model and P Controller q/4 -> Sum1/2
  Sum1/1 -> Bus Creator1/3  "Vey_err"
  Ref Model and P Controller q/3 -> Bus Creator1/2, Sum1/1  "Ve_y_sf"
  Ref Model and P Controller q/2 -> Bus Creator1/1  "Vey_sf_dot"
  Ref Model and P Controller p/5 -> Bus Creator/4  "K_b_Vex"
  Ref Model and P Controller p/4 -> Sum/2
  Selector2/1 -> Ref Model and P Controller r/2
  Bus Creator2/1 -> Terminator3/1
  Bus Creator1/1 -> Terminator1/1
  Bus Creator/1 -> Terminator2/1
  Sum/1 -> Bus Creator/3  "Vex_err"
  Ref Model and P Controller p/3 -> Bus Creator/2, Sum/1  "Vex_sf"
  Ref Model and P Controller p/2 -> Bus Creator/1  "Vex_sf_dot"
  Ref Model and P Controller r/1 -> Mux/3
  Ref Model and P Controller q/1 -> Mux/2
  Vyaw_z_ref/1 -> Ref Model and P Controller r/1
  Selector1/1 -> Ref Model and P Controller q/2
  Vyaw_y_ref/1 -> Ref Model and P Controller q/1
  Mux/1 -> Acc_yaw des (m/s)/1
  Ref Model and P Controller p/1 -> Mux/1
  Selector/1 -> Ref Model and P Controller p/2
  Vyaw_x_ref/1 -> Ref Model and P Controller p/1
  V_yaw_meas/1 -> Selector2/1, Selector1/1, Selector/1

== system Tricopter_Controlled_development/TriCopter FCS development/Outer Controller/Underactuated P Controller/Position Controller ==
  X_e_x_ref : Inport
  X_e_y_ref : Inport  Port=2
  X_e_z_ref : Inport  Port=3
  All_meas : Inport  Port=4
  Bus Creator : BusCreator
  Bus Creator1 : BusCreator
  Bus Creator2 : BusCreator
  Bus Selector : BusSelector  OutputSignals=Meas.Pos meas (m)
  Mux : Mux  Inputs=3
  Ref Model and P Controller p : Adaptive_FaultTolerantControl/Ref Model and P Controller  tau=5  y_i=0  K_f=0.5  K_b=1
  Ref Model and P Controller q : Adaptive_FaultTolerantControl/Ref Model and P Controller  tau=5  y_i=0  K_f=0.5  K_b=1
  Ref Model and P Controller r : Adaptive_FaultTolerantControl/Ref Model and P Controller  tau=5  y_i=-Alt_0  K_f=0.5  K_b=2
  Selector : Selector  InputPortWidth=3
  Selector1 : Selector  InputPortWidth=3  Indices=2
  Selector2 : Selector  InputPortWidth=3  Indices=3
  Sum : Sum  Inputs=+-|
  Sum1 : Sum  Inputs=+-|
  Sum2 : Sum  Inputs=+-|
  Terminator1 : Terminator
  Terminator2 : Terminator
  Terminator3 : Terminator
  Ve des (m/s) : Outport
  wires:
  Ref Model and P Controller r/5 -> Bus Creator2/4  "K_b_X_e_z"
  Ref Model and P Controller r/4 -> Sum2/2
  Sum2/1 -> Bus Creator2/3  "X_ez_err"
  Ref Model and P Controller r/3 -> Bus Creator2/2, Sum2/1  "X_ez_sf"
  Ref Model and P Controller r/2 -> Bus Creator2/1  "X_ez_sf_dot"
  Ref Model and P Controller q/5 -> Bus Creator1/4  "K_b_X_ey"
  Ref Model and P Controller q/4 -> Sum1/2
  Sum1/1 -> Bus Creator1/3  "X_ey_err"
  Ref Model and P Controller q/3 -> Bus Creator1/2, Sum1/1  "X_e_y_sf"
  Ref Model and P Controller q/2 -> Bus Creator1/1  "X_ey_sf_dot"
  Ref Model and P Controller p/5 -> Bus Creator/4  "K_b_X_ex"
  Ref Model and P Controller p/4 -> Sum/2
  Selector2/1 -> Ref Model and P Controller r/2
  Bus Creator2/1 -> Terminator3/1
  Bus Creator1/1 -> Terminator1/1
  Bus Creator/1 -> Terminator2/1
  Sum/1 -> Bus Creator/3  "X_ex_err"
  Ref Model and P Controller p/3 -> Bus Creator/2, Sum/1  "X_ex_sf"
  Ref Model and P Controller p/2 -> Bus Creator/1  "X_ex_sf_dot"
  Ref Model and P Controller r/1 -> Mux/3
  Ref Model and P Controller q/1 -> Mux/2
  X_e_z_ref/1 -> Ref Model and P Controller r/1
  Selector1/1 -> Ref Model and P Controller q/2
  X_e_y_ref/1 -> Ref Model and P Controller q/1
  Mux/1 -> Ve des (m/s)/1
  Ref Model and P Controller p/1 -> Mux/1
  Selector/1 -> Ref Model and P Controller p/2
  X_e_x_ref/1 -> Ref Model and P Controller p/1
  Bus Selector/1 -> Selector2/1, Selector1/1, Selector/1  "<Pos meas (m)>"
  All_meas/1 -> Bus Selector/1

== system Tricopter_Controlled_development/TriCopter FCS development/Outer Controller/Underactuated P Controller/Velocity Controller ==
  Ve_x_ref : Inport
  Ve_y_ref : Inport  Port=2
  Ve_z_ref : Inport  Port=3
  All_meas : Inport  Port=4
  Bus Creator : BusCreator
  Bus Creator1 : BusCreator
  Bus Creator2 : BusCreator
  Bus Selector : BusSelector  OutputSignals=Meas.V_e_meas
  Mux : Mux  Inputs=3
  Ref Model and P Controller p : Adaptive_FaultTolerantControl/Ref Model and P Controller  tau=2  y_i=0  K_f=0.5  K_b=1
  Ref Model and P Controller q : Adaptive_FaultTolerantControl/Ref Model and P Controller  tau=2  y_i=0  K_f=0.5  K_b=1
  Ref Model and P Controller r : Adaptive_FaultTolerantControl/Ref Model and P Controller  tau=2  y_i=0  K_f=0.5  K_b=1
  Selector : Selector  InputPortWidth=3
  Selector1 : Selector  InputPortWidth=3  Indices=2
  Selector2 : Selector  InputPortWidth=3  Indices=3
  Sum : Sum  Inputs=+-|
  Sum1 : Sum  Inputs=+-|
  Sum2 : Sum  Inputs=+-|
  Terminator1 : Terminator
  Terminator2 : Terminator
  Terminator3 : Terminator
  Acc_e des (m/s) : Outport
  wires:
  All_meas/1 -> Bus Selector/1
  Bus Selector/1 -> Selector/1, Selector1/1, Selector2/1  "<V_e_meas>"
  Ve_x_ref/1 -> Ref Model and P Controller p/1
  Selector/1 -> Ref Model and P Controller p/2
  Ref Model and P Controller p/1 -> Mux/1
  Mux/1 -> Acc_e des (m/s)/1
  Ve_y_ref/1 -> Ref Model and P Controller q/1
  Selector1/1 -> Ref Model and P Controller q/2
  Ve_z_ref/1 -> Ref Model and P Controller r/1
  Ref Model and P Controller q/1 -> Mux/2
  Ref Model and P Controller r/1 -> Mux/3
  Ref Model and P Controller p/2 -> Bus Creator/1  "Vex_sf_dot"
  Ref Model and P Controller p/3 -> Sum/1, Bus Creator/2  "Vex_sf"
  Sum/1 -> Bus Creator/3  "Vex_err"
  Bus Creator/1 -> Terminator2/1
  Bus Creator1/1 -> Terminator1/1
  Bus Creator2/1 -> Terminator3/1
  Selector2/1 -> Ref Model and P Controller r/2
  Ref Model and P Controller p/4 -> Sum/2
  Ref Model and P Controller p/5 -> Bus Creator/4  "K_b_Vex"
  Ref Model and P Controller q/2 -> Bus Creator1/1  "Vey_sf_dot"
  Ref Model and P Controller q/3 -> Sum1/1, Bus Creator1/2  "Ve_y_sf"
  Sum1/1 -> Bus Creator1/3  "Vey_err"
  Ref Model and P Controller q/4 -> Sum1/2
  Ref Model and P Controller q/5 -> Bus Creator1/4  "K_b_Vey"
  Ref Model and P Controller r/2 -> Bus Creator2/1  "Vez_sf_dot"
  Ref Model and P Controller r/3 -> Sum2/1, Bus Creator2/2  "Vez_sf"
  Sum2/1 -> Bus Creator2/3  "Vez_err"
  Ref Model and P Controller r/4 -> Sum2/2
  Ref Model and P Controller r/5 -> Bus Creator2/4  "K_b_Ve_z"

== system Tricopter_Controlled_development/FlightGear visualization/Flat Earth to LLA/ne to lat//long/LongLat_offset /Find Radian//Distance  ==
  note: R
  mu : Inport
  Constant{,2..3,5..6} (5 alike) : Constant
  Constant1 : Constant  Value=6378137
  Constant4 : Constant  Value=1/298.257223563
  Product1 : Product  Inputs=*/  RndMeth=Zero
  Product2 : Product  RndMeth=Zero
  Product3 : Product  Inputs=**/  RndMeth=Zero
  Product4 : Product  RndMeth=Zero
  Product5 : Product  RndMeth=Zero
  Product6 : Product  Inputs=4  RndMeth=Zero
  Sum : Sum  Inputs=-+
  Sum1 : Sum  Inputs=|+-
  Sum2 : Sum  Inputs=|+-
  Sum3 : Sum  Inputs=|+-
  Trigonometric Function : Trigonometry  Operator=cos
  Trigonometric Function1 : Trigonometry  Operator=atan2
  Trigonometric Function2 : Trigonometry  Operator=atan2
  Trigonometric Function3 : Trigonometry
  deg2rad : Gain  Gain=pi/180  SaturateOnIntegerOverflow=on  OutDataTypeStr=Inherit: Same as input  ParamDataTypeStr=Inherit: Same as input
  f : Constant
  sqrt : Sqrt  AlgorithmType=Newton-Raphson  SaturateOnIntegerOverflow=on
  sqrt1 : Sqrt  AlgorithmType=Newton-Raphson  SaturateOnIntegerOverflow=on
  dNorth : Outport
  dEast : Outport  Port=2
  wires:
  Trigonometric Function2/1 -> dEast/1
  Trigonometric Function1/1 -> dNorth/1
  Constant3/1 -> Trigonometric Function2/1
  Constant2/1 -> Trigonometric Function1/1
  Product4/1 -> Trigonometric Function2/2
  mu/1 -> deg2rad/1
  Trigonometric Function/1 -> Product4/2
  Product3/1 -> Trigonometric Function1/2  "Rm"
  Sum1/1 -> Product3/2
  Product1/1 -> Product4/1, Product3/1  "Rn"
  Constant/1 -> Sum1/1
  Product2/1 -> Sum1/2
  Constant1/1 -> Product1/1
  sqrt/1 -> Product1/2
  Sum3/1 -> Product3/3, sqrt/1
  f/1 -> Sum/2
  Constant4/1 -> Sum/1
  Sum/1 -> Product5/1, Product5/2
  Product5/1 -> Sum2/2
  Constant5/1 -> Sum2/1
  Sum2/1 -> sqrt1/1
  deg2rad/1 -> Trigonometric Function3/1, Trigonometric Function/1
  Trigonometric Function3/1 -> Product6/4, Product6/3
  sqrt1/1 -> Product6/1, Product6/2, Product2/2, Product2/1
  Product6/1 -> Sum3/2
  Constant6/1 -> Sum3/1

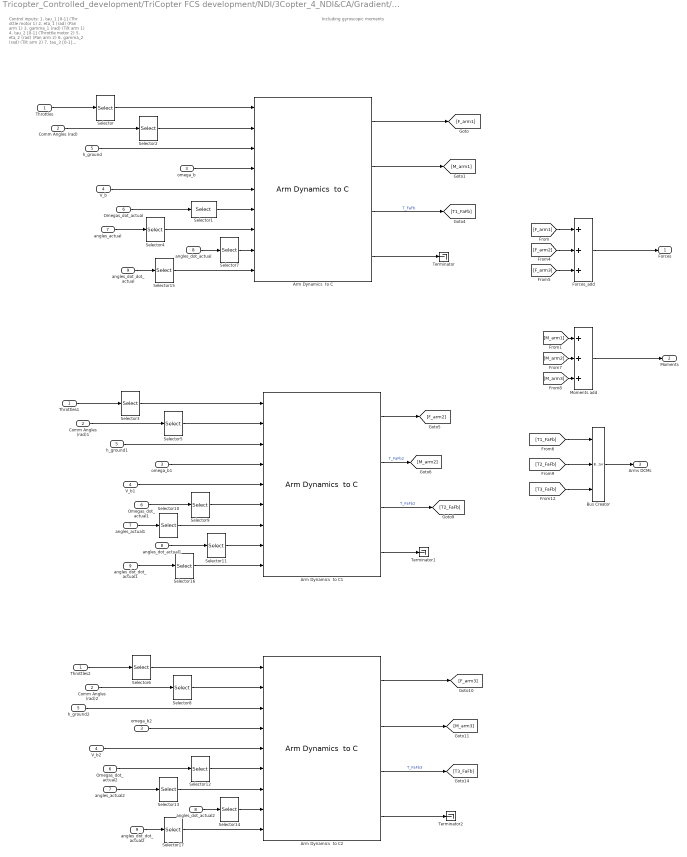
== system Tricopter_Controlled_development/TriCopter FCS development/NDI/3Copter_4_NDI&CA/Gradient/Arms Dynamics: Forces and Moments ==
  note: Including gyroscopic moments
  note: Control inputs:
      | 1. tau_1 [0-1] (Thr ottle motor 1)
      | 2. eta_1 (rad)  (Pan arm 1)
      | 3. gamma_1 (rad)  (Tilt arm 1)
      |
      | 4. tau_2 [0-1] (Throttle motor 2)
      | 5. eta_2 (rad)  (Pan arm 2)
      | 6. gamma_2 (rad)  (Tilt arm 2)
      |
      | 7. tau_3 [0-1] (Throttle motor 3)
      | 8. eta_3 (rad)  (Pan arm  3)
      | 9. gamma_3 (rad)  (Tilt arm 3)
  Throttles : Inport
  Comm Angles (rad) : Inport  Port=2
  omega_b : Inport  Port=3
  V_b : Inport  Port=4
  h_ground : Inport  Port=5
  Omegas_dot_actual : Inport  Port=6
  angles_actual : Inport  Port=7
  angles_dot_actual : Inport  Port=8
  angles_dot_dot_actual : Inport  Port=9
  Arm Dynamics  to C : XXCopter_Control/Arm Dynamics  to C  Rot_sign=Rotation_sign(1)  arm_hub_pos=l*[1;0;0]  Arm_axis=[l_arm;0;0]  arm_num=1  eta_dir=[1;0;0]  gamma_dir=[0;1;0]  J_T=J_T  J_FA=J_FA  h=h  switch_val=direct_feedforward  omega_n=30  xi=1.4  eta_inf_lim=deg2rad(-180)  eta_sup_lim=deg2rad(180)  gamma_inf_lim=deg2rad(-90)  gamma_sup_lim=deg2rad(15)
  Arm Dynamics  to C1 : XXCopter_Control/Arm Dynamics  to C  Rot_sign=Rotation_sign(2)  arm_hub_pos=l*[-1/2;sqrt(3)/2;0]  Arm_axis=[0;l_arm;0]  arm_num=2  eta_dir=[0;1;0]  gamma_dir=[1;0;0]  J_T=J_T  J_FA=J_FA  h=h  switch_val=direct_feedforward  omega_n=30  xi=1.4  eta_inf_lim=deg2rad(-180)  eta_sup_lim=deg2rad(180)  gamma_inf_lim=deg2rad(-15)  gamma_sup_lim=deg2rad(90)
  Arm Dynamics  to C2 : XXCopter_Control/Arm Dynamics  to C  Rot_sign=Rotation_sign(3)  arm_hub_pos=l*[-1/2;-sqrt(3)/2;0]  Arm_axis=[0;-l_arm;0]  arm_num=3  eta_dir=[0;1;0]  gamma_dir=[1;0;0]  J_T=J_T  J_FA=J_FA  h=h  switch_val=direct_feedforward  omega_n=30  xi=1.4  eta_inf_lim=deg2rad(-180)  eta_sup_lim=deg2rad(180)  gamma_inf_lim=deg2rad(-90)  gamma_sup_lim=deg2rad(15)
  Bus Creator : BusCreator  Inputs=3
  Comm Angles (rad)1 : InportShadow  Port=2
  Comm Angles (rad)2 : InportShadow  Port=2
  Forces_add : Sum  Inputs=+++
  Moments add : Sum  Inputs=+++
  Omegas_dot_actual1 : InportShadow  Port=6
  Omegas_dot_actual2 : InportShadow  Port=6
  Selector : Selector  IndexMode=Zero-based  InputPortWidth=3  Indices=0
  Selector1 : Selector  IndexMode=Zero-based  InputPortWidth=3  Indices=0
  Selector{5,10..11,16} (4 alike) : Selector  IndexMode=Zero-based  InputPortWidth=6  Indices=[2,3]
  Selector12 : Selector  IndexMode=Zero-based  InputPortWidth=3  Indices=2
  Selector{8,13..14,17} (4 alike) : Selector  IndexMode=Zero-based  InputPortWidth=6  Indices=[4,5]
  Selector{2,4,7,15} (4 alike) : Selector  IndexMode=Zero-based  InputPortWidth=6  Indices=[0,1]
  Selector3 : Selector  IndexMode=Zero-based  InputPortWidth=3
  Selector6 : Selector  IndexMode=Zero-based  InputPortWidth=3  Indices=2
  Selector9 : Selector  IndexMode=Zero-based  InputPortWidth=3
  Terminator : Terminator
  Terminator1 : Terminator
  Terminator2 : Terminator
  Throttles1 : InportShadow
  Throttles2 : InportShadow
  V_b1 : InportShadow  Port=4
  V_b2 : InportShadow  Port=4
  angles_actual1 : InportShadow  Port=7
  angles_actual2 : InportShadow  Port=7
  angles_dot_actual1 : InportShadow  Port=8
  angles_dot_actual2 : InportShadow  Port=8
  angles_dot_dot_actual1 : InportShadow  Port=9
  angles_dot_dot_actual2 : InportShadow  Port=9
  h_ground1 : InportShadow  Port=5
  h_ground2 : InportShadow  Port=5
  omega_b1 : InportShadow  Port=3
  omega_b2 : InportShadow  Port=3
  Forces : Outport
  Moments : Outport  Port=2
  Arms DCMs : Outport  Port=3
  wires:
  Selector14/1 -> Arm Dynamics  to C2/8
  angles_actual2/1 -> Selector13/1
  angles_dot_actual2/1 -> Selector14/1
  Selector13/1 -> Arm Dynamics  to C2/7
  Selector12/1 -> Arm Dynamics  to C2/6
  Omegas_dot_actual2/1 -> Selector12/1
  Selector11/1 -> Arm Dynamics  to C1/8
  angles_actual1/1 -> Selector10/1
  angles_dot_actual1/1 -> Selector11/1
  Selector10/1 -> Arm Dynamics  to C1/7
  Selector9/1 -> Arm Dynamics  to C1/6
  Omegas_dot_actual1/1 -> Selector9/1
  Selector7/1 -> Arm Dynamics  to C/8
  angles_dot_actual/1 -> Selector7/1
  Selector4/1 -> Arm Dynamics  to C/7
  angles_actual/1 -> Selector4/1
  Selector1/1 -> Arm Dynamics  to C/6
  Omegas_dot_actual/1 -> Selector1/1
  [T3_FaFb] -> Bus Creator/3
  [T2_FaFb] -> Bus Creator/2
  [T1_FaFb] -> Bus Creator/1
  Bus Creator/1 -> Arms DCMs/1
  Arm Dynamics  to C1/2 -> [M_arm2]  "T_FaFb2"
  Arm Dynamics  to C1/1 -> [F_arm2]
  Arm Dynamics  to C2/4 -> Terminator2/1
  Arm Dynamics  to C1/4 -> Terminator1/1
  Arm Dynamics  to C/4 -> Terminator/1
  Arm Dynamics  to C2/3 -> [T3_FaFb]  "T_FaFb3"
  Comm Angles (rad)2/1 -> Selector8/1
  Selector8/1 -> Arm Dynamics  to C2/2
  omega_b2/1 -> Arm Dynamics  to C2/4
  Arm Dynamics  to C2/2 -> [M_arm3]
  Arm Dynamics  to C2/1 -> [F_arm3]
  h_ground2/1 -> Arm Dynamics  to C2/3
  V_b2/1 -> Arm Dynamics  to C2/5
  Selector6/1 -> Arm Dynamics  to C2/1
  Throttles2/1 -> Selector6/1
  Arm Dynamics  to C1/3 -> [T2_FaFb]  "T_FaFb2"
  Comm Angles (rad)1/1 -> Selector5/1
  Selector5/1 -> Arm Dynamics  to C1/2
  omega_b1/1 -> Arm Dynamics  to C1/4
  h_ground1/1 -> Arm Dynamics  to C1/3
  V_b1/1 -> Arm Dynamics  to C1/5
  Selector3/1 -> Arm Dynamics  to C1/1
  Throttles1/1 -> Selector3/1
  Arm Dynamics  to C/3 -> [T1_FaFb]  "T_FaFb"
  Comm Angles (rad)/1 -> Selector2/1
  Selector2/1 -> Arm Dynamics  to C/2
  [M_arm2] -> Moments add/2
  [M_arm3] -> Moments add/3
  [F_arm3] -> Forces_add/3
  [F_arm2] -> Forces_add/2
  omega_b/1 -> Arm Dynamics  to C/4
  [M_arm1] -> Moments add/1
  [F_arm1] -> Forces_add/1
  Arm Dynamics  to C/2 -> [M_arm1]
  Arm Dynamics  to C/1 -> [F_arm1]
  h_ground/1 -> Arm Dynamics  to C/3
  Moments add/1 -> Moments/1
  Forces_add/1 -> Forces/1
  V_b/1 -> Arm Dynamics  to C/5
  Selector/1 -> Arm Dynamics  to C/1
  Throttles/1 -> Selector/1
  angles_dot_dot_actual/1 -> Selector15/1
  Selector15/1 -> Arm Dynamics  to C/9
  angles_dot_dot_actual1/1 -> Selector16/1
  Selector16/1 -> Arm Dynamics  to C1/9
  angles_dot_dot_actual2/1 -> Selector17/1
  Selector17/1 -> Arm Dynamics  to C2/9

== matlab function Tricopter_Controlled_development/3 Copter Complete/6dof Eqs of motion/Position Eqs ==
  data: A_b output; Vb input; omega input; omega_dot input; Forces input; m input; CG input
function A_b  = PositionEqs(Vb,omega,omega_dot, Forces,m, CG)



 
A_b =  1/m*( Forces ) - cross(omega,Vb) - cross(omega, cross(omega,CG)) -cross(omega_dot,CG)  ;

== matlab function Tricopter_Controlled_development/3 Copter Complete/6dof Eqs of motion/Rotational eqs ==
  data: omega_dot output; omega_b input; Moments input; I_BAC input
function omega_dot  = Rotational_Eq(omega_b,Moments, I_BAC)



omega_dot =  I_BAC\( Moments - cross(omega_b,I_BAC*omega_b)  );

== matlab function Tricopter_Controlled_development/3 Copter Complete/6dof Eqs of motion/q_dot/Quaternion_dot ==
  data: omega_b input; q_dot output; q input
function q_dot = Quaternion_dot(omega_b,q)


q_dot = 1/2*HamiltonProduct(q,[0;omega_b]);

function Product= HamiltonProduct( a,b )

Product=[ a(1)*b(1)-a(2)*b(2)-a(3)*b(3)-a(4)*b(4) ; a(1)*b(2)+a(2)*b(1)+a(3)*b(4)-a(4)*b(3)  ; a(1)*b(3)-a(2)*b(4)+a(3)*b(1)+a(4)*b(2)  ; a(1)*b(4)+a(2)*b(3)-a(3)*b(2)+a(4)*b(1) ];

== matlab function Tricopter_Controlled_development/3 Copter Complete/Gravity Force and Moment ==
  data: q input; F_g_b output; M_g_b output; mass input; CG input; g parameter
function [F_g_b,M_g_b]   = Grav_Forces_and_Mom( q,mass,CG, g)

Prod=HamiltonProduct([q(1);-q(2);-q(3);-q(4)],HamiltonProduct([0;0;0;mass*g],[q(1);q(2);q(3);q(4)]) ); % q* . g .q

F_g_b= Prod(2:4);
M_g_b=cross(CG,F_g_b);

function Product= HamiltonProduct( a,b )

Product=[ a(1)*b(1)-a(2)*b(2)-a(3)*b(3)-a(4)*b(4) ; a(1)*b(2)+a(2)*b(1)+a(3)*b(4)-a(4)*b(3)  ; a(1)*b(3)-a(2)*b(4)+a(3)*b(1)+a(4)*b(2)  ; a(1)*b(4)+a(2)*b(3)-a(3)*b(2)+a(4)*b(1) ];

== matlab function Tricopter_Controlled_development/3 Copter Complete/Aerodynamics body Force and Moment1 ==
  data: V_b input; F_a_b output; M_a_b output; rho parameter; C_x parameter; C_y parameter; C_z parameter; A_x parameter; A_y parameter; A_z parameter
function [F_a_b,M_a_b]   = Aero_body_Forces_and_Mom( V_b, rho,C_x,C_y,C_z,A_x,A_y,A_z)


F_a_b=1/2*rho*(V_b*V_b')*[C_x*A_x;C_y*A_y;C_z*A_z].*( - V_b./(norm(V_b)+eps) );
M_a_b=[0;0;0];
end

== matlab function Tricopter_Controlled_development/3 Copter Complete/6dof Eqs of motion/Eccelerometer meas ==
  data: Vb input; omega input; omega_dot input; Ab input; A_s output; r_sens parameter
function A_s  = AcellMeas(Vb,omega,omega_dot,Ab, r_sens)




A_s =  Ab + cross(omega,Vb) + cross(omega, cross(omega,r_sens)) +cross(omega_dot,r_sens)  ;

== matlab function Tricopter_Controlled_development/3 Copter Complete/6dof Eqs of motion/SVFI_to_SVFb ==
  data: X_e input; V_e input; X_e_out output; V_b output; omega_b output; Euler_Ang input; Euler_Ang_Dot input; q output
function [X_e_out,V_b, omega_b ,q]=SVFI_to_SVFb(X_e,V_e, Euler_Ang,Euler_Ang_Dot)

q = zeros(4,1);
V_b =zeros(3,1);

xp=V_e(1);
yp=V_e(2);
zp=V_e(3);

phi=Euler_Ang(1);
theta=Euler_Ang(2);
psi=Euler_Ang(3);
phip=Euler_Ang_Dot(1);
thetap=Euler_Ang_Dot(2);
psip=Euler_Ang_Dot(3);

%%
X_e_out=X_e;

q = QuaternionfromEuler(phi,theta,psi); 



HamOut=HamiltonProduct([q(1);-q(2);-q(3);-q(4)],HamiltonProduct([0;xp;yp;zp],[q(1);q(2);q(3);q(4)]) );% q* . v . q
V_b=HamOut(2:4);

omega_b=[phip-psip*sin(theta)  ;
         thetap*cos(phi)+psip*cos(theta)*sin(phi);
            -thetap*sin(phi)+psip*cos(theta)*cos(phi)  ];% Ya que es solo una operacion aislada utilizaremos la ecuaciones con rel trigonometricas

function [q]=QuaternionfromEuler(phi,theta,psi)
% options=optimset('MaxFunEvals',3000);
% q=fsolve(@QUATERNIONEULER,[0.6,0.4,0.5,0.4]); % Hay que acertar con los angulos poniendo diferentes valores iniciales del quaternion
%     function F=QUATERNIONEULER(q)
%         F=[ tan(phi)-(2*q(3)*q(4)-2*q(1)*q(2))/(2*q(1)^2+2*q(4)^2-1)  ;
%             sin(-theta)-2*q(2)*q(4)-2*q(1)*q(3);
%             tan(psi)-(2*q(2)*q(3)-2*q(1)*q(4))/(2*q(1)^2+2*q(2)^2-1);
%             q(1)^2+q(2)^2+q(3)^2+q(4)^2-1];
%     end  % Este algoritmo da q* !!!!!

q=[ cos(psi/2)*cos(theta/2)*cos(phi/2)+ sin(psi/2)*sin(theta/2)*sin(phi/2) ;
      cos(psi/2)*cos(theta/2)*sin(phi/2)- sin(psi/2)*sin(theta/2)*cos(phi/2) ;
       cos(psi/2)*sin(theta/2)*cos(phi/2)+ sin(psi/2)*cos(theta/2)*sin(phi/2)   ;
        sin(psi/2)*cos(theta/2)*cos(phi/2)- cos(psi/2)*sin(theta/2)*sin(phi/2)      ]; % Esto nos da q !!!

    function Product= HamiltonProduct( a,b )

Product=[ a(1)*b(1)-a(2)*b(2)-a(3)*b(3)-a(4)*b(4) ; a(1)*b(2)+a(2)*b(1)+a(3)*b(4)-a(4)*b(3)  ; a(1)*b(3)-a(2)*b(4)+a(3)*b(1)+a(4)*b(2)  ; a(1)*b(4)+a(2)*b(3)-a(3)*b(2)+a(4)*b(1) ];

== matlab function Tricopter_Controlled_development/3 Copter Complete/6dof Eqs of motion/SV_F_b_to_SV_FI ==
  data: V_b input; q_dot input; q input; V_e output; euler output; euler_dot output
function [V_e,euler,euler_dot]   = SV_F_b_to_SV_FI(  V_b, q_dot,q)

xp=V_b(1);
yp=V_b(2);
zp=V_b(3);

%% Velocity and position in Earth Frame   q . v . q*

SolProd=HamiltonProduct([q(1);q(2);q(3);q(4)],HamiltonProduct([0;xp;yp;zp],[q(1);-q(2);-q(3);-q(4)]) );
V_e=SolProd(2:4);

%% Actitud en Angulos de Euler y sus derivadas. 
euler=[0,0,0]';
euler(1,1) = atan2(2*q(3)*q(4)+2*q(1)*q(2),2*q(1)^2+2*q(4)^2-1 ); % phi
euler(2,1) = -asin( 2*q(2)*q(4)-2*q(1)*q(3) ); %  theta
euler(3,1) = atan2( 2*q(2)*q(3)+2*q(1)*q(4),2*q(1)^2+2*q(2)^2-1 ); %  psi

euler_dot=[0,0,0]';
euler_dot(1,1) = 2/(1+( (2*q(3)*q(4)+2*q(1)*q(2))/(2*q(1)^2+2*q(4)^2-1)  )^2)*[ -(2*q(1)^2*q(2)+ 4*q(1)*q(3)*q(4)-2*q(2)*q(4)^2+q(2))  ,  q(1)*(2*q(1)^2+2*q(4)^2-1)  ,  q(4)*(2*q(1)^2+2*q(4)^2-1)  ,  -(-2*q(1)^2*q(3) +4*q(1)*q(2)*q(4)+2*q(3)*q(4)^2+q(3) ) ]*q_dot.* 1/(2*q(1)^2+2*q(4)^2-1)^2; % Derivada de phi
euler_dot(2,1) = -2/( sqrt(1-4*(q(2)*q(4)-q(1)*q(3))^2)  )*[-q(3),q(4),-q(1),q(2)]*q_dot;  % Theta prima
euler_dot(3,1) = 2/(1+( (2*q(2)*q(3)+2*q(1)*q(4))/(2*q(1)^2+2*q(2)^2-1)  )^2)*[  -(2*q(1)^2*q(4)+4*q(1)*q(2)*q(3)-2*q(2)^2*q(4)+q(4)  ) , 1/2*(q(3)*(4*q(1)^2-4*q(2)^2-2)-8*q(1)*q(2)*q(4) )  ,  q(2)*(2*q(1)^2+2*q(2)^2-1)  , q(1)*(2*q(1)^2+2*q(2)^2-1) ]*q_dot.*1/(2*q(1)^2+2*q(2)^2-1)^2;  % Psi prima


function Product= HamiltonProduct( a,b )

Product=[ a(1)*b(1)-a(2)*b(2)-a(3)*b(3)-a(4)*b(4) ; a(1)*b(2)+a(2)*b(1)+a(3)*b(4)-a(4)*b(3)  ; a(1)*b(3)-a(2)*b(4)+a(3)*b(1)+a(4)*b(2)  ; a(1)*b(4)+a(2)*b(3)-a(3)*b(2)+a(4)*b(1) ];

== matlab function Tricopter_Controlled_development/3 Copter Complete/Mass Properties/Arm Inertia ==
  data: T1_FAFb input; T2_FAFb input; T3_FAFb input; I_M output; l parameter; h_M parameter; m_M parameter; r1_M output; r2_M output; r3_M output
function [I_M,r1_M,r2_M,r3_M]  = Arm1_inertia(T1_FAFb,T2_FAFb,T3_FAFb, l, h_M, m_M)


r1_M=[l;0;0]+T1_FAFb*[0;0;-h_M];
r2_M=[-1/2*l;sqrt(3)/2*l;0]+T2_FAFb*[0;0;-h_M];
r3_M=[-1/2*l;-sqrt(3)/2*l;0]+T3_FAFb*[0;0;-h_M];


I_M1 = m_M*[ r1_M(2)^2+r1_M(3)^2,r1_M(1)*r1_M(2),r1_M(1)*r1_M(3);...
            r1_M(1)*r1_M(2), r1_M(1)^2+r1_M(3)^2, r1_M(2)*r1_M(3);...
            r1_M(1)*r1_M(3),r1_M(2)*r1_M(3), r1_M(1)^2+r1_M(2)^2];
I_M2 = m_M*[ r2_M(2)^2+r2_M(3)^2,r2_M(1)*r2_M(2),r2_M(1)*r2_M(3);...
            r2_M(1)*r2_M(2), r2_M(1)^2+r2_M(3)^2, r2_M(2)*r2_M(3);...
            r2_M(1)*r2_M(3),r2_M(2)*r2_M(3), r2_M(1)^2+r2_M(2)^2];
I_M3 = m_M*[ r3_M(2)^2+r3_M(3)^2,r3_M(1)*r3_M(2),r3_M(1)*r3_M(3);...
            r3_M(1)*r3_M(2), r3_M(1)^2+r3_M(3)^2, r3_M(2)*r3_M(3);...
            r3_M(1)*r3_M(3),r3_M(2)*r3_M(3), r3_M(1)^2+r3_M(2)^2];

I_M = I_M1+I_M2+I_M3;

== matlab function Tricopter_Controlled_development/TriCopter FCS development/Inner Controller/P Controller/MATLAB Function ==
  data: ang_dot input size=[3,1]; Omega output; euler_ang input size=[3,1]
function Omega = Euler_dot_2_omega(ang_dot,euler_ang)

phi = euler_ang(1);
theta = euler_ang(2);
psi = euler_ang(3);


A = [1  0 -sin(theta);
     0       cos(phi)         sin(phi)*cos(theta);
     0  -sin(phi)   cos(phi)*cos(theta)];

Omega = A*ang_dot ;

== matlab function Tricopter_Controlled_development/TriCopter FCS development/Inner Controller/PI Controller/Limits in Ang accel/Limis eval ==
  data: Ang_Accel input size=[3,1]; Limit_up output; euler_ang input size=[3,1]; Limit_down output; l parameter; m parameter; g parameter; A_l_max_x parameter; Ix parameter; Iy parameter; Iz parameter
function [Limit_up,Limit_down]= Max_ang_accels(Ang_Accel,euler_ang,l,m,g,A_l_max_x,Ix,Iy,Iz)

Limit_up=Ang_Accel;
Limit_down=Ang_Accel;

Limit_up(1) = max(   abs( (2*m*g/3*sqrt(3)/2*l  )/Ix*cos(euler_ang(1))   ), abs(  2/3*A_l_max_x*sqrt(3)/2*l/Ix*sin(euler_ang(2)) ) )* 0.5 ;
Limit_down(1) = -Limit_up(1) ;

Limit_up(2) = max(  (l*m*g*2/3-l/2*m*g/3)/Iy*cos(euler_ang(2)) , (2*l*A_l_max_x)/Iy*sin(euler_ang(2)) )* 0.5 ;
Limit_down(2) = - max( (l/2*m*g)/Iy*cos(euler_ang(2))  , (2*l*A_l_max_x)/Iy*sin(euler_ang(2)) )* 0.5 ;


Limit_up(3) = max(  abs(  A_l_max_x*l/Iz*cos(euler_ang(1))*cos(euler_ang(2)) ) , abs(  (2*m*g/3*sqrt(3)/2*l  )/Iz*sin(euler_ang(2)) )  )* 0.5 ;
Limit_down(3) = -Limit_up(1) ;
